simulink model "fft_test"  (R2019a)
settings: Solver=VariableStepDiscrete  StartTime=0.0  StopTime=50000  RelTol=1e-3
libraries: xbsIndex_r4 x4228, casper_library_misc x129, xps_library x1
(part 1 of 42)
settings Model: Creator=cicada  LastModifiedBy=kocz
settings SolverCC: ZeroCrossControl=EnableAll
settings DataIOCC: LimitDataPoints=on  SaveFormat=Array  SignalLoggingSaveFormat=ModelDataLogs  ReturnWorkspaceOutputs=off
settings OptimizationCC: DefaultParameterBehavior=Inlined  ExpressionDepthLimit=2147483647  LifeSpan=inf
settings DebuggingCC: WriteAfterWriteMsg=EnableAllAsError  SignalResolutionControl=TryResolveAllWithWarning  SolverPrmCheckMsg=warning  FcnCallInpInsideContextMsg=warning  StateNameClashWarn=warning  PregeneratedLibrarySubsystemCodeDiagnostic=none  StrictBusMsg=ErrorOnBusTreatedAsVector  SFUnexpectedBacktrackingDiag=warning  SFNoUnconditionalDefaultTransitionDiag=warning  SFExecutionAtInitializationDiag=none  ArithmeticOperatorsInVariantConditions=warning
settings HardwareCC: ProdBitPerPointer=32  ProdBitPerSizeT=32  ProdBitPerPtrDiffT=32  ProdLargestAtomicFloat=None  ProdIntDivRoundTo=Undefined  ProdEndianess=Unspecified  ProdWordSize=32  ProdHWDeviceType=32-bit Generic
settings ModelReferenceCC: PropagateSignalLabelsOutOfModel=off
settings SFSimCC: SimUseLocalCustomCode=off
settings RTWCC: RTWUseLocalCustomCode=off
settings CodeAppCC: StateflowObjectComments=on
settings GRTTargetCC: TargetLangStandard=C89/C90 (ANSI)  GeneratePreprocessorConditionals=Disable all  CombineOutputUpdateFcns=off  GRTInterface=on
settings ConfigComp: CovMetricSettings=dw  CovHtmlReporting=on  CovSaveCumulativeToWorkspaceVar=on  CovSaveSingleToWorkspaceVar=on  CovExternalEMLEnable=off

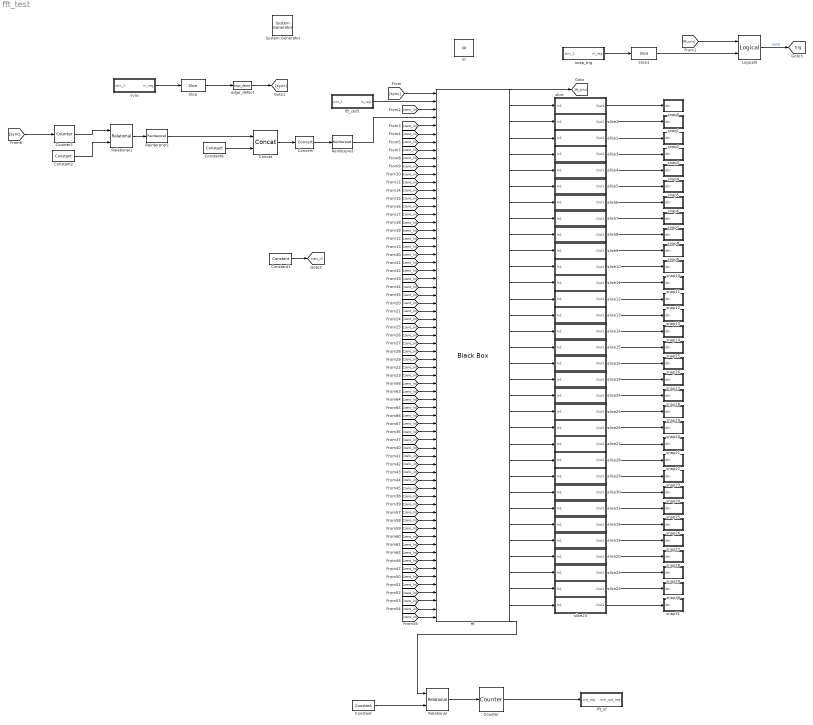
== system fft_test ==
  " System Generator" : xbsIndex_r4/ System Generator  Tag=genX  xilinxfamily=kintex7  part=xc7k325t  speed=-3  package=fbg676  synthesis_tool=Vivado  clock_wrapper=Clock Enables  directory=./netlist  proj_type=Vivado  Synth_file=Vivado Synthesis Defaults  Impl_file=Vivado Implementation Defaults  testbench=off  simulink_period=1  sysclk_period=10  dcm_input_clock_period=10  incr_netlist=off  trim_vbits=Everywhere in SubSystem  dbl_ovrd=According to Block Masks  core_generation=According to Block Masks  run_coregen=off  deprecated_control=off  eval_field=0  block_type=sysgen
  Concat : xbsIndex_r4/Concat  num_inputs=2  dbl_ovrd=off  block_type=concat
  Constant : xbsIndex_r4/Constant  const=0  gui_display_data_type=Fixed-point  arith_type=Unsigned  n_bits=16  bin_pt=0  preci_type=Single  exp_width=8  frac_width=24  explicit_period=on  period=1  equ=P=C  opselect=C  inp2=PCIN>>17  opr=+  inp1=P  carry=CIN  dbl_ovrd=off  block_type=constant
  Constant1 : xbsIndex_r4/Constant  const=0  gui_display_data_type=Fixed-point  arith_type=Signed (2's comp)  n_bits=18  bin_pt=17  preci_type=Single  exp_width=8  frac_width=24  explicit_period=on  period=1  equ=P=C  opselect=C  inp2=PCIN>>17  opr=+  inp1=P  carry=CIN  dbl_ovrd=off  block_type=constant
  Constant2 : xbsIndex_r4/Constant  const=1  gui_display_data_type=Fixed-point  arith_type=Unsigned  n_bits=32  bin_pt=0  preci_type=Single  exp_width=8  frac_width=24  explicit_period=on  period=1  equ=P=C  opselect=C  inp2=PCIN>>17  opr=+  inp1=P  carry=CIN  dbl_ovrd=off  block_type=constant
  Constant6 : xbsIndex_r4/Constant  const=0  gui_display_data_type=Fixed-point  arith_type=Unsigned  n_bits=4  bin_pt=0  preci_type=Single  exp_width=8  frac_width=24  explicit_period=on  period=1  equ=P=C  opselect=C  inp2=PCIN>>17  opr=+  inp1=P  carry=CIN  dbl_ovrd=off  block_type=constant
  Convert : xbsIndex_r4/Convert  gui_display_data_type=Fixed-point  arith_type=Unsigned  n_bits=18  bin_pt=0  float_type=Single  exp_bits=8  fraction_bits=24  quantization=Truncate  overflow=Wrap  en=off  latency=2  pipeline=off  dbl_ovrd=off  block_type=convert
  Counter : xbsIndex_r4/Counter  cnt_type=Free Running  cnt_to=Inf  operation=Up  start_count=0  cnt_by_val=1  arith_type=Unsigned  n_bits=16  bin_pt=0  load_pin=off  rst=off  en=on  explicit_period=on  period=1  use_behavioral_HDL=off  implementation=Fabric  dbl_ovrd=off  block_type=counter
  Counter1 : xbsIndex_r4/Counter  cnt_type=Free Running  cnt_to=Inf  operation=Up  start_count=0  cnt_by_val=1  arith_type=Unsigned  n_bits=12  bin_pt=0  load_pin=off  rst=on  en=off  explicit_period=on  period=1  use_behavioral_HDL=off  implementation=Fabric  dbl_ovrd=off  block_type=counter
  Logical5 : xbsIndex_r4/Logical  logical_function=AND  inputs=2  en=off  latency=1  precision=Full  arith_type=Unsigned  n_bits=16  bin_pt=0  align_bp=on  dbl_ovrd=off  block_type=logical
  Reinterpret : xbsIndex_r4/Reinterpret  force_arith_type=on  arith_type="Signed  (2's comp)"  force_bin_pt=on  bin_pt=17  block_type=reinterpret
  Reinterpret1 : xbsIndex_r4/Reinterpret  force_arith_type=on  arith_type=Unsigned  force_bin_pt=on  bin_pt=0  block_type=reinterpret
  Relational : xbsIndex_r4/Relational  mode=a>b  op_type=Bool  en=off  latency=1  dbl_ovrd=off  block_type=relational
  Relational1 : xbsIndex_r4/Relational  mode=a=b  op_type=Bool  en=off  latency=0  dbl_ovrd=off  block_type=relational
  Slice : xbsIndex_r4/Slice  nbits=1  boolean_output=on  mode=Lower Bit Location + Width  bit1=0  base1=MSB of Input  bit0=0  base0=LSB of Input  dbl_ovrd=off  block_type=slice
  Slice1 : xbsIndex_r4/Slice  nbits=1  boolean_output=on  mode=Lower Bit Location + Width  bit1=0  base1=MSB of Input  bit0=0  base0=LSB of Input  dbl_ovrd=off  block_type=slice
  edge_detect : casper_library_misc/edge_detect  edge=Rising  polarity=Active High  x_in=[0 0.08 0.08 0.16 0.16 0.24 0.24 0.32 0.32 0.4]  y_in="[-1 -1  1  1  1  1  1  1  1  1]"  x_out=[0.6 0.68 0.68 0.76 0.76 0.84 0.84 0.92 0.92 1]  y_out="[-1 -1  1  1 -1 -1 -1 -1 -1 -1]"
  fft : xbsIndex_r4/Black Box  init_code=fft_2019_rord_config  sim_method=ISE Simulator  verbose=off  block_type=blackbox2
  fft_of : Subsystem  Tag=xps:sw_reg  AncestorBlock=xps_library/Memory/software_register  mask(swreg){io_dir=To Processor, io_delay=0, init_val=0, sample_period=1, names=reg, bitwidths=16, bin_pts=0, arith_types=0, sim_port=on, show_format=on}
      mask prompts: io_dir "I/O direction"; io_delay "I/O delay"; init_val "Initial Value"; sample_period "Sample period"; names "Bitfield names [msb...lsb]"; bitwidths "Bitfield widths"; bin_pts "Bitfield binary pts"; arith_types "Bitfield types, ufix=0, fix=1, bool=2"; sim_port "Provide sim input/output?"; show_format "Print format string?"
      mask help: A 32-bit software-accessible register. Can be divided into bitfields of varying widths and types using the fields in the block mask.
      mask init:
      | swreg_init(gcb)
      settings: AttributesFormatString=1output:uf16.0 = 16 bits
      mask TypeOptions io_dir: To Processor | From Processor
      mask Callback io_dir:
      | mask_enables = get_param(gcb, 'MaskEnables');
      | mask_names = get_param(gcb, 'MaskNames');
      | if strcmp(get_param(gcb, 'io_dir'), 'To Processor'),
      |     mask_enables{ismember(mask_names, 'sample_period')} = 'off';
      | else
      |     mask_enables{ismember(mask_names, 'sample_period')} = 'on';
      | end
      | set_param(gcb, 'MaskEnables', mask_enables);
      mask DialogControl ParameterTabVar0 Prompt: Setup
  fft_shift : Subsystem  Tag=xps:sw_reg  AncestorBlock=xps_library/Memory/software_register  mask(swreg){io_dir=From Processor, io_delay=0, init_val=0, sample_period=1, names=reg, bitwidths=32, bin_pts=0, arith_types=0, sim_port=on, show_format=on}
      mask prompts: io_dir "I/O direction"; io_delay "I/O delay"; init_val "Initial Value"; sample_period "Sample period"; names "Bitfield names [msb...lsb]"; bitwidths "Bitfield widths"; bin_pts "Bitfield binary pts"; arith_types "Bitfield types, ufix=0, fix=1, bool=2"; sim_port "Provide sim input/output?"; show_format "Print format string?"
      mask help: A 32-bit software-accessible register. Can be divided into bitfields of varying widths and types using the fields in the block mask.
      mask init:
      | swreg_init(gcb)
      settings: AttributesFormatString=1input:uf32.0 = 32 bits
      mask TypeOptions io_dir: To Processor | From Processor
      mask Callback io_dir:
      | mask_enables = get_param(gcb, 'MaskEnables');
      | mask_names = get_param(gcb, 'MaskNames');
      | if strcmp(get_param(gcb, 'io_dir'), 'To Processor'),
      |     mask_enables{ismember(mask_names, 'sample_period')} = 'off';
      | else
      |     mask_enables{ismember(mask_names, 'sample_period')} = 'on';
      | end
      | set_param(gcb, 'MaskEnables', mask_enables);
      mask DialogControl ParameterTabVar0 Prompt: Setup
  ip : xps_library/Utilities/ip  Tag=xps:ip  lib_path=[fileparts(which(gcs)) '/fft_2019_default']  ip_name='fft_2019_default'
      settings: SourceProductName=CASPER XPS Blockset
  slice : Subsystem
  slice1 : Subsystem
  slice10 : Subsystem
  slice11 : Subsystem
  slice12 : Subsystem
  slice13 : Subsystem
  slice14 : Subsystem
  slice15 : Subsystem
  slice16 : Subsystem
  slice17 : Subsystem
  slice18 : Subsystem
  slice19 : Subsystem
  slice2 : Subsystem
  slice20 : Subsystem
  slice21 : Subsystem
  slice22 : Subsystem
  slice23 : Subsystem
  slice24 : Subsystem
  slice25 : Subsystem
  slice26 : Subsystem
  slice27 : Subsystem
  slice28 : Subsystem
  slice29 : Subsystem
  slice3 : Subsystem
  slice30 : Subsystem
  slice31 : Subsystem
  slice4 : Subsystem
  slice5 : Subsystem
  slice6 : Subsystem
  slice7 : Subsystem
  slice8 : Subsystem
  slice9 : Subsystem
  snap0 : Subsystem
  snap1 : Subsystem
  snap10 : Subsystem
  snap11 : Subsystem
  snap12 : Subsystem
  snap13 : Subsystem
  snap14 : Subsystem
  snap15 : Subsystem
  snap16 : Subsystem
  snap17 : Subsystem
  snap18 : Subsystem
  snap19 : Subsystem
  snap2 : Subsystem
  snap20 : Subsystem
  snap21 : Subsystem
  snap22 : Subsystem
  snap23 : Subsystem
  snap24 : Subsystem
  snap25 : Subsystem
  snap26 : Subsystem
  snap27 : Subsystem
  snap28 : Subsystem
  snap29 : Subsystem
  snap3 : Subsystem
  snap30 : Subsystem
  snap31 : Subsystem
  snap4 : Subsystem
  snap5 : Subsystem
  snap6 : Subsystem
  snap7 : Subsystem
  snap8 : Subsystem
  snap9 : Subsystem
  snap_trig : Subsystem  Tag=xps:sw_reg  AncestorBlock=xps_library/Memory/software_register  mask(swreg){io_dir=From Processor, io_delay=0, init_val=0, sample_period=1, names=reg, bitwidths=32, bin_pts=0, arith_types=0, sim_port=on, show_format=on}
      mask prompts: io_dir "I/O direction"; io_delay "I/O delay"; init_val "Initial Value"; sample_period "Sample period"; names "Bitfield names [msb...lsb]"; bitwidths "Bitfield widths"; bin_pts "Bitfield binary pts"; arith_types "Bitfield types, ufix=0, fix=1, bool=2"; sim_port "Provide sim input/output?"; show_format "Print format string?"
      mask help: A 32-bit software-accessible register. Can be divided into bitfields of varying widths and types using the fields in the block mask.
      mask init:
      | swreg_init(gcb)
      settings: AttributesFormatString=1input:uf32.0 = 32 bits
      mask TypeOptions io_dir: To Processor | From Processor
      mask Callback io_dir:
      | mask_enables = get_param(gcb, 'MaskEnables');
      | mask_names = get_param(gcb, 'MaskNames');
      | if strcmp(get_param(gcb, 'io_dir'), 'To Processor'),
      |     mask_enables{ismember(mask_names, 'sample_period')} = 'off';
      | else
      |     mask_enables{ismember(mask_names, 'sample_period')} = 'on';
      | end
      | set_param(gcb, 'MaskEnables', mask_enables);
      mask DialogControl ParameterTabVar0 Prompt: Setup
  sync : Subsystem  Tag=xps:sw_reg  AncestorBlock=xps_library/Memory/software_register  mask(swreg){io_dir=From Processor, io_delay=0, init_val=0, sample_period=1, names=reg, bitwidths=32, bin_pts=0, arith_types=0, sim_port=on, show_format=on}
      mask prompts: io_dir "I/O direction"; io_delay "I/O delay"; init_val "Initial Value"; sample_period "Sample period"; names "Bitfield names [msb...lsb]"; bitwidths "Bitfield widths"; bin_pts "Bitfield binary pts"; arith_types "Bitfield types, ufix=0, fix=1, bool=2"; sim_port "Provide sim input/output?"; show_format "Print format string?"
      mask help: A 32-bit software-accessible register. Can be divided into bitfields of varying widths and types using the fields in the block mask.
      mask init:
      | swreg_init(gcb)
      settings: AttributesFormatString=1input:uf32.0 = 32 bits
      mask TypeOptions io_dir: To Processor | From Processor
      mask Callback io_dir:
      | mask_enables = get_param(gcb, 'MaskEnables');
      | mask_names = get_param(gcb, 'MaskNames');
      | if strcmp(get_param(gcb, 'io_dir'), 'To Processor'),
      |     mask_enables{ismember(mask_names, 'sample_period')} = 'off';
      | else
      |     mask_enables{ismember(mask_names, 'sample_period')} = 'on';
      | end
      | set_param(gcb, 'MaskEnables', mask_enables);
      mask DialogControl ParameterTabVar0 Prompt: Setup
  tag scope: trig=global
  wires:
  fft_shift/1(in_reg) -> fft/2
  fft/1 -> [fft_sync]
  Relational/1 -> Counter/1
  Constant/1 -> Relational/2
  fft/34 -> Relational/1
  Counter/1 -> fft_of/1(out_reg)
  Slice/1 -> edge_detect/1
  sync/1(in_reg) -> Slice/1
  Constant6/1 -> Concat/2
  Reinterpret1/1 -> Concat/1
  Relational1/1 -> Reinterpret1/1
  Concat/1 -> Convert/1
  Convert/1 -> Reinterpret/1
  Constant2/1 -> Relational1/2
  Counter1/1 -> Relational1/1
  Reinterpret/1 -> fft/4
  edge_detect/1 -> [sync]
  Constant1/1 -> [zero_in]
  [zero_in] -> fft/3
  [zero_in] -> fft/5
  [zero_in] -> fft/6
  [zero_in] -> fft/7
  [sync] -> fft/1
  [sync] -> Counter1/1
  [zero_in] -> fft/8
  [zero_in] -> fft/12
  [zero_in] -> fft/11
  [zero_in] -> fft/10
  [zero_in] -> fft/9
  [zero_in] -> fft/17
  [zero_in] -> fft/18
  [zero_in] -> fft/19
  [zero_in] -> fft/20
  [zero_in] -> fft/16
  [zero_in] -> fft/15
  [zero_in] -> fft/14
  [zero_in] -> fft/13
  [zero_in] -> fft/29
  [zero_in] -> fft/30
  [zero_in] -> fft/31
  [zero_in] -> fft/32
  [zero_in] -> fft/36
  [zero_in] -> fft/35
  [zero_in] -> fft/34
  [zero_in] -> fft/33
  [zero_in] -> fft/25
  [zero_in] -> fft/26
  [zero_in] -> fft/27
  [zero_in] -> fft/28
  [zero_in] -> fft/24
  [zero_in] -> fft/23
  [zero_in] -> fft/22
  [zero_in] -> fft/21
  [zero_in] -> fft/53
  [zero_in] -> fft/54
  [zero_in] -> fft/55
  [zero_in] -> fft/56
  [zero_in] -> fft/60
  [zero_in] -> fft/59
  [zero_in] -> fft/58
  [zero_in] -> fft/57
  [zero_in] -> fft/65
  [zero_in] -> fft/66
  [zero_in] -> fft/64
  [zero_in] -> fft/63
  [zero_in] -> fft/62
  [zero_in] -> fft/61
  [zero_in] -> fft/45
  [zero_in] -> fft/46
  [zero_in] -> fft/47
  [zero_in] -> fft/48
  [zero_in] -> fft/52
  [zero_in] -> fft/51
  [zero_in] -> fft/50
  [zero_in] -> fft/49
  [zero_in] -> fft/41
  [zero_in] -> fft/42
  [zero_in] -> fft/43
  [zero_in] -> fft/44
  [zero_in] -> fft/40
  [zero_in] -> fft/39
  [zero_in] -> fft/38
  [zero_in] -> fft/37
  fft/2 -> slice/1(In1)
  fft/3 -> slice1/1(In1)
  fft/4 -> slice2/1(In1)
  fft/5 -> slice3/1(In1)
  fft/6 -> slice4/1(In1)
  fft/7 -> slice5/1(In1)
  fft/8 -> slice6/1(In1)
  fft/9 -> slice7/1(In1)
  fft/10 -> slice8/1(In1)
  fft/11 -> slice9/1(In1)
  fft/12 -> slice10/1(In1)
  fft/13 -> slice11/1(In1)
  fft/14 -> slice12/1(In1)
  fft/15 -> slice13/1(In1)
  fft/16 -> slice14/1(In1)
  fft/17 -> slice15/1(In1)
  fft/18 -> slice16/1(In1)
  fft/19 -> slice17/1(In1)
  fft/20 -> slice24/1(In1)
  fft/21 -> slice25/1(In1)
  fft/22 -> slice26/1(In1)
  fft/23 -> slice27/1(In1)
  fft/24 -> slice28/1(In1)
  fft/25 -> slice29/1(In1)
  fft/26 -> slice30/1(In1)
  fft/27 -> slice31/1(In1)
  fft/28 -> slice18/1(In1)
  fft/29 -> slice19/1(In1)
  fft/30 -> slice20/1(In1)
  fft/31 -> slice21/1(In1)
  fft/32 -> slice22/1(In1)
  fft/33 -> slice23/1(In1)
  slice/1(Out1) -> snap0/1(din)
  slice1/1(Out1) -> snap1/1(din)
  slice3/1(Out1) -> snap3/1(din)
  slice2/1(Out1) -> snap2/1(din)
  slice5/1(Out1) -> snap5/1(din)
  slice7/1(Out1) -> snap7/1(din)
  slice6/1(Out1) -> snap6/1(din)
  slice4/1(Out1) -> snap4/1(din)
  slice12/1(Out1) -> snap12/1(din)
  slice11/1(Out1) -> snap11/1(din)
  slice15/1(Out1) -> snap15/1(din)
  slice8/1(Out1) -> snap8/1(din)
  slice9/1(Out1) -> snap9/1(din)
  slice13/1(Out1) -> snap13/1(din)
  slice10/1(Out1) -> snap10/1(din)
  slice14/1(Out1) -> snap14/1(din)
  slice18/1(Out1) -> snap26/1(din)
  slice16/1(Out1) -> snap16/1(din)
  slice27/1(Out1) -> snap21/1(din)
  slice21/1(Out1) -> snap29/1(din)
  slice28/1(Out1) -> snap22/1(din)
  slice29/1(Out1) -> snap23/1(din)
  slice26/1(Out1) -> snap20/1(din)
  slice22/1(Out1) -> snap30/1(din)
  slice23/1(Out1) -> snap31/1(din)
  slice31/1(Out1) -> snap25/1(din)
  slice25/1(Out1) -> snap19/1(din)
  slice30/1(Out1) -> snap24/1(din)
  slice17/1(Out1) -> snap17/1(din)
  slice20/1(Out1) -> snap28/1(din)
  slice19/1(Out1) -> snap27/1(din)
  slice24/1(Out1) -> snap18/1(din)
  [fft_sync] -> Logical5/1
  snap_trig/1(in_reg) -> Slice1/1
  Slice1/1 -> Logical5/2
  Logical5/1 -> [trig]  "valid"

== system fft_test/fft_of ==
  out_reg : Inport
  assert_reg : xbsIndex_r4/Assert  assert_type=on  type_source=Explicitly  gui_display_data_type=Fixed-point  arith_type=Unsigned  n_bits=16  bin_pt=0  preci_type=Single  exp_width=8  frac_width=24  assert_rate=off  rate_source=Explicitly  period=1  output_port=on  block_type=assert
  cast_gw : xbsIndex_r4/Convert  gui_display_data_type=Fixed-point  arith_type=Unsigned  n_bits=32  bin_pt=0  float_type=Single  exp_bits=8  fraction_bits=24  quantization=Truncate  overflow=Wrap  en=off  latency=1  pipeline=off  dbl_ovrd=off  block_type=convert
  fft_test_fft_of_user_data_in : xbsIndex_r4/Gateway Out  inherit_from_input=off  hdl_port=on  rows=1  columns=1  UseAsDAC=off  DACChannel='1'  interface=None  automatic_assignment=on  address_offset=hex2dec('00')  intf_name=''  intf_description=''  timing_constraint=None  locs_specified=off  LOCs={}  io_standard={}  block_type=gatewayout
  io_delay : xbsIndex_r4/Delay  rst=off  infoeditControl=Selection of Reset will increase slice count due to use of real FFs and instead of SRLs  en=off  latency=0  reg_retiming=on  dbl_ovrd=off  block_type=delay
  reint1 : xbsIndex_r4/Reinterpret  force_arith_type=on  arith_type=Unsigned  force_bin_pt=on  bin_pt=0  block_type=reinterpret
  sim_out : Terminator
  sim_out_reg_gw : xbsIndex_r4/Gateway Out  inherit_from_input=off  hdl_port=off  rows=1  columns=1  UseAsDAC=off  DACChannel='1'  interface=None  automatic_assignment=on  address_offset=hex2dec('00')  intf_name=''  intf_description=''  timing_constraint=None  locs_specified=off  LOCs={}  io_standard={}  block_type=gatewayout
  sim_out_reg_sim_delay : xbsIndex_r4/Delay  rst=off  infoeditControl=Selection of Reset will increase slice count due to use of real FFs and instead of SRLs  en=off  latency=1  reg_retiming=on  dbl_ovrd=off  block_type=delay
  sim_out_reg : Outport
  wires:
  sim_out_reg_sim_delay/1 -> sim_out_reg_gw/1
  sim_out_reg_gw/1 -> sim_out_reg/1
  io_delay/1 -> cast_gw/1
  cast_gw/1 -> fft_test_fft_of_user_data_in/1
  fft_test_fft_of_user_data_in/1 -> sim_out/1
  out_reg/1 -> sim_out_reg_sim_delay/1, assert_reg/1
  assert_reg/1 -> reint1/1
  reint1/1 -> io_delay/1

== system fft_test/fft_shift ==
  sim_1 : Inport
  convert1_1 : DataTypeConversion  OutDataTypeStr=fixdt('ufix32_En0')  LockScale=on
  convert2_1 : DataTypeConversion  OutDataTypeStr=fixdt('ufix32_En0')  ConvertRealWorld=Stored Integer (SI)  LockScale=on
  fft_test_fft_shift_user_data_out : xbsIndex_r4/Gateway In  gui_display_data_type=Fixed-point  arith_type=Unsigned  n_bits=32  bin_pt=0  preci_type=Single  exp_width=8  frac_width=24  rows=1  columns=1  quantization="Round  (unbiased: +/- Inf)"  overflow=Saturate  period=1  UseAsADC=off  ADCChannel='1'  interface=None  automatic_assignment=on  address_offset=hex2dec('00')  intf_name=''  intf_description=''  default_value=0  timing_constraint=None  locs_specified=off  LOCs={}  io_standard={}  inherit_from_input=off  hdl_port=on  dbl_ovrd=off  block_type=gatewayin
  gain_1 : Gain
  io_delay : xbsIndex_r4/Delay  rst=off  infoeditControl=Selection of Reset will increase slice count due to use of real FFs and instead of SRLs  en=off  latency=0  reg_retiming=on  dbl_ovrd=off  block_type=delay
  reint1 : xbsIndex_r4/Reinterpret  force_arith_type=on  arith_type=Unsigned  force_bin_pt=on  bin_pt=0  block_type=reinterpret
  slice_reg : xbsIndex_r4/Slice  nbits=32  boolean_output=off  mode=Lower Bit Location + Width  bit1=0  base1=MSB of Input  bit0=0  base0=LSB of Input  dbl_ovrd=off  block_type=slice
  in_reg : Outport
  wires:
  fft_test_fft_shift_user_data_out/1 -> io_delay/1
  sim_1/1 -> convert1_1/1
  convert1_1/1 -> convert2_1/1
  convert2_1/1 -> gain_1/1
  gain_1/1 -> fft_test_fft_shift_user_data_out/1
  io_delay/1 -> slice_reg/1
  slice_reg/1 -> reint1/1
  reint1/1 -> in_reg/1

== system fft_test/slice ==
  In1 : Inport
  Slice1 : xbsIndex_r4/Slice  nbits=16  boolean_output=off  mode=Upper Bit Location + Width  bit1=0  base1=MSB of Input  bit0=0  base0=LSB of Input  dbl_ovrd=off  block_type=slice
  Slice2 : xbsIndex_r4/Slice  nbits=16  boolean_output=off  mode=Upper Bit Location + Width  bit1=0  base1=MSB of Input  bit0=0  base0=LSB of Input  dbl_ovrd=off  block_type=slice
  c_to_ri : casper_library_misc/c_to_ri  n_bits=8  bin_pt=7
      settings: AttributesFormatString=8_7 r/i  SourceProductName=CASPER DSP Blockset
  ri_to_c : casper_library_misc/ri_to_c
      settings: SourceProductName=CASPER DSP Blockset
  Out1 : Outport
  wires:
  Slice1/1 -> ri_to_c/1
  In1/1 -> c_to_ri/1
  Slice2/1 -> ri_to_c/2
  c_to_ri/1 -> Slice1/1
  ri_to_c/1 -> Out1/1
  c_to_ri/2 -> Slice2/1

== system fft_test/slice1 ==
  In1 : Inport
  Slice1 : xbsIndex_r4/Slice  nbits=16  boolean_output=off  mode=Upper Bit Location + Width  bit1=0  base1=MSB of Input  bit0=0  base0=LSB of Input  dbl_ovrd=off  block_type=slice
  Slice2 : xbsIndex_r4/Slice  nbits=16  boolean_output=off  mode=Upper Bit Location + Width  bit1=0  base1=MSB of Input  bit0=0  base0=LSB of Input  dbl_ovrd=off  block_type=slice
  c_to_ri : casper_library_misc/c_to_ri  n_bits=8  bin_pt=7
      settings: AttributesFormatString=8_7 r/i  SourceProductName=CASPER DSP Blockset
  ri_to_c : casper_library_misc/ri_to_c
      settings: SourceProductName=CASPER DSP Blockset
  Out1 : Outport
  wires:
  c_to_ri/2 -> Slice2/1
  ri_to_c/1 -> Out1/1
  c_to_ri/1 -> Slice1/1
  Slice2/1 -> ri_to_c/2
  In1/1 -> c_to_ri/1
  Slice1/1 -> ri_to_c/1

== system fft_test/slice10 ==
  In1 : Inport
  Slice1 : xbsIndex_r4/Slice  nbits=16  boolean_output=off  mode=Upper Bit Location + Width  bit1=0  base1=MSB of Input  bit0=0  base0=LSB of Input  dbl_ovrd=off  block_type=slice
  Slice2 : xbsIndex_r4/Slice  nbits=16  boolean_output=off  mode=Upper Bit Location + Width  bit1=0  base1=MSB of Input  bit0=0  base0=LSB of Input  dbl_ovrd=off  block_type=slice
  c_to_ri : casper_library_misc/c_to_ri  n_bits=8  bin_pt=7
      settings: AttributesFormatString=8_7 r/i  SourceProductName=CASPER DSP Blockset
  ri_to_c : casper_library_misc/ri_to_c
      settings: SourceProductName=CASPER DSP Blockset
  Out1 : Outport
  wires:
  Slice1/1 -> ri_to_c/1
  In1/1 -> c_to_ri/1
  Slice2/1 -> ri_to_c/2
  c_to_ri/1 -> Slice1/1
  ri_to_c/1 -> Out1/1
  c_to_ri/2 -> Slice2/1

== system fft_test/slice11 ==
  In1 : Inport
  Slice1 : xbsIndex_r4/Slice  nbits=16  boolean_output=off  mode=Upper Bit Location + Width  bit1=0  base1=MSB of Input  bit0=0  base0=LSB of Input  dbl_ovrd=off  block_type=slice
  Slice2 : xbsIndex_r4/Slice  nbits=16  boolean_output=off  mode=Upper Bit Location + Width  bit1=0  base1=MSB of Input  bit0=0  base0=LSB of Input  dbl_ovrd=off  block_type=slice
  c_to_ri : casper_library_misc/c_to_ri  n_bits=8  bin_pt=7
      settings: AttributesFormatString=8_7 r/i  SourceProductName=CASPER DSP Blockset
  ri_to_c : casper_library_misc/ri_to_c
      settings: SourceProductName=CASPER DSP Blockset
  Out1 : Outport
  wires:
  c_to_ri/2 -> Slice2/1
  ri_to_c/1 -> Out1/1
  c_to_ri/1 -> Slice1/1
  Slice2/1 -> ri_to_c/2
  In1/1 -> c_to_ri/1
  Slice1/1 -> ri_to_c/1

== system fft_test/slice12 ==
  In1 : Inport
  Slice1 : xbsIndex_r4/Slice  nbits=16  boolean_output=off  mode=Upper Bit Location + Width  bit1=0  base1=MSB of Input  bit0=0  base0=LSB of Input  dbl_ovrd=off  block_type=slice
  Slice2 : xbsIndex_r4/Slice  nbits=16  boolean_output=off  mode=Upper Bit Location + Width  bit1=0  base1=MSB of Input  bit0=0  base0=LSB of Input  dbl_ovrd=off  block_type=slice
  c_to_ri : casper_library_misc/c_to_ri  n_bits=8  bin_pt=7
      settings: AttributesFormatString=8_7 r/i  SourceProductName=CASPER DSP Blockset
  ri_to_c : casper_library_misc/ri_to_c
      settings: SourceProductName=CASPER DSP Blockset
  Out1 : Outport
  wires:
  Slice1/1 -> ri_to_c/1
  In1/1 -> c_to_ri/1
  Slice2/1 -> ri_to_c/2
  c_to_ri/1 -> Slice1/1
  ri_to_c/1 -> Out1/1
  c_to_ri/2 -> Slice2/1

== system fft_test/slice13 ==
  In1 : Inport
  Slice1 : xbsIndex_r4/Slice  nbits=16  boolean_output=off  mode=Upper Bit Location + Width  bit1=0  base1=MSB of Input  bit0=0  base0=LSB of Input  dbl_ovrd=off  block_type=slice
  Slice2 : xbsIndex_r4/Slice  nbits=16  boolean_output=off  mode=Upper Bit Location + Width  bit1=0  base1=MSB of Input  bit0=0  base0=LSB of Input  dbl_ovrd=off  block_type=slice
  c_to_ri : casper_library_misc/c_to_ri  n_bits=8  bin_pt=7
      settings: AttributesFormatString=8_7 r/i  SourceProductName=CASPER DSP Blockset
  ri_to_c : casper_library_misc/ri_to_c
      settings: SourceProductName=CASPER DSP Blockset
  Out1 : Outport
  wires:
  c_to_ri/2 -> Slice2/1
  ri_to_c/1 -> Out1/1
  c_to_ri/1 -> Slice1/1
  Slice2/1 -> ri_to_c/2
  In1/1 -> c_to_ri/1
  Slice1/1 -> ri_to_c/1

== system fft_test/slice14 ==
  In1 : Inport
  Slice1 : xbsIndex_r4/Slice  nbits=16  boolean_output=off  mode=Upper Bit Location + Width  bit1=0  base1=MSB of Input  bit0=0  base0=LSB of Input  dbl_ovrd=off  block_type=slice
  Slice2 : xbsIndex_r4/Slice  nbits=16  boolean_output=off  mode=Upper Bit Location + Width  bit1=0  base1=MSB of Input  bit0=0  base0=LSB of Input  dbl_ovrd=off  block_type=slice
  c_to_ri : casper_library_misc/c_to_ri  n_bits=8  bin_pt=7
      settings: AttributesFormatString=8_7 r/i  SourceProductName=CASPER DSP Blockset
  ri_to_c : casper_library_misc/ri_to_c
      settings: SourceProductName=CASPER DSP Blockset
  Out1 : Outport
  wires:
  c_to_ri/2 -> Slice2/1
  ri_to_c/1 -> Out1/1
  c_to_ri/1 -> Slice1/1
  Slice2/1 -> ri_to_c/2
  In1/1 -> c_to_ri/1
  Slice1/1 -> ri_to_c/1

== system fft_test/slice15 ==
  In1 : Inport
  Slice1 : xbsIndex_r4/Slice  nbits=16  boolean_output=off  mode=Upper Bit Location + Width  bit1=0  base1=MSB of Input  bit0=0  base0=LSB of Input  dbl_ovrd=off  block_type=slice
  Slice2 : xbsIndex_r4/Slice  nbits=16  boolean_output=off  mode=Upper Bit Location + Width  bit1=0  base1=MSB of Input  bit0=0  base0=LSB of Input  dbl_ovrd=off  block_type=slice
  c_to_ri : casper_library_misc/c_to_ri  n_bits=8  bin_pt=7
      settings: AttributesFormatString=8_7 r/i  SourceProductName=CASPER DSP Blockset
  ri_to_c : casper_library_misc/ri_to_c
      settings: SourceProductName=CASPER DSP Blockset
  Out1 : Outport
  wires:
  Slice1/1 -> ri_to_c/1
  In1/1 -> c_to_ri/1
  Slice2/1 -> ri_to_c/2
  c_to_ri/1 -> Slice1/1
  ri_to_c/1 -> Out1/1
  c_to_ri/2 -> Slice2/1

== system fft_test/slice16 ==
  In1 : Inport
  Slice1 : xbsIndex_r4/Slice  nbits=16  boolean_output=off  mode=Upper Bit Location + Width  bit1=0  base1=MSB of Input  bit0=0  base0=LSB of Input  dbl_ovrd=off  block_type=slice
  Slice2 : xbsIndex_r4/Slice  nbits=16  boolean_output=off  mode=Upper Bit Location + Width  bit1=0  base1=MSB of Input  bit0=0  base0=LSB of Input  dbl_ovrd=off  block_type=slice
  c_to_ri : casper_library_misc/c_to_ri  n_bits=8  bin_pt=7
      settings: AttributesFormatString=8_7 r/i  SourceProductName=CASPER DSP Blockset
  ri_to_c : casper_library_misc/ri_to_c
      settings: SourceProductName=CASPER DSP Blockset
  Out1 : Outport
  wires:
  c_to_ri/2 -> Slice2/1
  ri_to_c/1 -> Out1/1
  c_to_ri/1 -> Slice1/1
  Slice2/1 -> ri_to_c/2
  In1/1 -> c_to_ri/1
  Slice1/1 -> ri_to_c/1

== system fft_test/slice17 ==
  In1 : Inport
  Slice1 : xbsIndex_r4/Slice  nbits=16  boolean_output=off  mode=Upper Bit Location + Width  bit1=0  base1=MSB of Input  bit0=0  base0=LSB of Input  dbl_ovrd=off  block_type=slice
  Slice2 : xbsIndex_r4/Slice  nbits=16  boolean_output=off  mode=Upper Bit Location + Width  bit1=0  base1=MSB of Input  bit0=0  base0=LSB of Input  dbl_ovrd=off  block_type=slice
  c_to_ri : casper_library_misc/c_to_ri  n_bits=8  bin_pt=7
      settings: AttributesFormatString=8_7 r/i  SourceProductName=CASPER DSP Blockset
  ri_to_c : casper_library_misc/ri_to_c
      settings: SourceProductName=CASPER DSP Blockset
  Out1 : Outport
  wires:
  Slice1/1 -> ri_to_c/1
  In1/1 -> c_to_ri/1
  Slice2/1 -> ri_to_c/2
  c_to_ri/1 -> Slice1/1
  ri_to_c/1 -> Out1/1
  c_to_ri/2 -> Slice2/1

== system fft_test/slice18 ==
  In1 : Inport
  Slice1 : xbsIndex_r4/Slice  nbits=16  boolean_output=off  mode=Upper Bit Location + Width  bit1=0  base1=MSB of Input  bit0=0  base0=LSB of Input  dbl_ovrd=off  block_type=slice
  Slice2 : xbsIndex_r4/Slice  nbits=16  boolean_output=off  mode=Upper Bit Location + Width  bit1=0  base1=MSB of Input  bit0=0  base0=LSB of Input  dbl_ovrd=off  block_type=slice
  c_to_ri : casper_library_misc/c_to_ri  n_bits=8  bin_pt=7
      settings: AttributesFormatString=8_7 r/i  SourceProductName=CASPER DSP Blockset
  ri_to_c : casper_library_misc/ri_to_c
      settings: SourceProductName=CASPER DSP Blockset
  Out1 : Outport
  wires:
  c_to_ri/2 -> Slice2/1
  ri_to_c/1 -> Out1/1
  c_to_ri/1 -> Slice1/1
  Slice2/1 -> ri_to_c/2
  In1/1 -> c_to_ri/1
  Slice1/1 -> ri_to_c/1

== system fft_test/slice19 ==
  In1 : Inport
  Slice1 : xbsIndex_r4/Slice  nbits=16  boolean_output=off  mode=Upper Bit Location + Width  bit1=0  base1=MSB of Input  bit0=0  base0=LSB of Input  dbl_ovrd=off  block_type=slice
  Slice2 : xbsIndex_r4/Slice  nbits=16  boolean_output=off  mode=Upper Bit Location + Width  bit1=0  base1=MSB of Input  bit0=0  base0=LSB of Input  dbl_ovrd=off  block_type=slice
  c_to_ri : casper_library_misc/c_to_ri  n_bits=8  bin_pt=7
      settings: AttributesFormatString=8_7 r/i  SourceProductName=CASPER DSP Blockset
  ri_to_c : casper_library_misc/ri_to_c
      settings: SourceProductName=CASPER DSP Blockset
  Out1 : Outport
  wires:
  Slice1/1 -> ri_to_c/1
  In1/1 -> c_to_ri/1
  Slice2/1 -> ri_to_c/2
  c_to_ri/1 -> Slice1/1
  ri_to_c/1 -> Out1/1
  c_to_ri/2 -> Slice2/1

== system fft_test/slice2 ==
  In1 : Inport
  Slice1 : xbsIndex_r4/Slice  nbits=16  boolean_output=off  mode=Upper Bit Location + Width  bit1=0  base1=MSB of Input  bit0=0  base0=LSB of Input  dbl_ovrd=off  block_type=slice
  Slice2 : xbsIndex_r4/Slice  nbits=16  boolean_output=off  mode=Upper Bit Location + Width  bit1=0  base1=MSB of Input  bit0=0  base0=LSB of Input  dbl_ovrd=off  block_type=slice
  c_to_ri : casper_library_misc/c_to_ri  n_bits=8  bin_pt=7
      settings: AttributesFormatString=8_7 r/i  SourceProductName=CASPER DSP Blockset
  ri_to_c : casper_library_misc/ri_to_c
      settings: SourceProductName=CASPER DSP Blockset
  Out1 : Outport
  wires:
  c_to_ri/2 -> Slice2/1
  ri_to_c/1 -> Out1/1
  c_to_ri/1 -> Slice1/1
  Slice2/1 -> ri_to_c/2
  In1/1 -> c_to_ri/1
  Slice1/1 -> ri_to_c/1

== system fft_test/slice20 ==
  In1 : Inport
  Slice1 : xbsIndex_r4/Slice  nbits=16  boolean_output=off  mode=Upper Bit Location + Width  bit1=0  base1=MSB of Input  bit0=0  base0=LSB of Input  dbl_ovrd=off  block_type=slice
  Slice2 : xbsIndex_r4/Slice  nbits=16  boolean_output=off  mode=Upper Bit Location + Width  bit1=0  base1=MSB of Input  bit0=0  base0=LSB of Input  dbl_ovrd=off  block_type=slice
  c_to_ri : casper_library_misc/c_to_ri  n_bits=8  bin_pt=7
      settings: AttributesFormatString=8_7 r/i  SourceProductName=CASPER DSP Blockset
  ri_to_c : casper_library_misc/ri_to_c
      settings: SourceProductName=CASPER DSP Blockset
  Out1 : Outport
  wires:
  c_to_ri/2 -> Slice2/1
  ri_to_c/1 -> Out1/1
  c_to_ri/1 -> Slice1/1
  Slice2/1 -> ri_to_c/2
  In1/1 -> c_to_ri/1
  Slice1/1 -> ri_to_c/1

== system fft_test/slice21 ==
  In1 : Inport
  Slice1 : xbsIndex_r4/Slice  nbits=16  boolean_output=off  mode=Upper Bit Location + Width  bit1=0  base1=MSB of Input  bit0=0  base0=LSB of Input  dbl_ovrd=off  block_type=slice
  Slice2 : xbsIndex_r4/Slice  nbits=16  boolean_output=off  mode=Upper Bit Location + Width  bit1=0  base1=MSB of Input  bit0=0  base0=LSB of Input  dbl_ovrd=off  block_type=slice
  c_to_ri : casper_library_misc/c_to_ri  n_bits=8  bin_pt=7
      settings: AttributesFormatString=8_7 r/i  SourceProductName=CASPER DSP Blockset
  ri_to_c : casper_library_misc/ri_to_c
      settings: SourceProductName=CASPER DSP Blockset
  Out1 : Outport
  wires:
  Slice1/1 -> ri_to_c/1
  In1/1 -> c_to_ri/1
  Slice2/1 -> ri_to_c/2
  c_to_ri/1 -> Slice1/1
  ri_to_c/1 -> Out1/1
  c_to_ri/2 -> Slice2/1

== system fft_test/slice22 ==
  In1 : Inport
  Slice1 : xbsIndex_r4/Slice  nbits=16  boolean_output=off  mode=Upper Bit Location + Width  bit1=0  base1=MSB of Input  bit0=0  base0=LSB of Input  dbl_ovrd=off  block_type=slice
  Slice2 : xbsIndex_r4/Slice  nbits=16  boolean_output=off  mode=Upper Bit Location + Width  bit1=0  base1=MSB of Input  bit0=0  base0=LSB of Input  dbl_ovrd=off  block_type=slice
  c_to_ri : casper_library_misc/c_to_ri  n_bits=8  bin_pt=7
      settings: AttributesFormatString=8_7 r/i  SourceProductName=CASPER DSP Blockset
  ri_to_c : casper_library_misc/ri_to_c
      settings: SourceProductName=CASPER DSP Blockset
  Out1 : Outport
  wires:
  Slice1/1 -> ri_to_c/1
  In1/1 -> c_to_ri/1
  Slice2/1 -> ri_to_c/2
  c_to_ri/1 -> Slice1/1
  ri_to_c/1 -> Out1/1
  c_to_ri/2 -> Slice2/1

== system fft_test/slice23 ==
  In1 : Inport
  Slice1 : xbsIndex_r4/Slice  nbits=16  boolean_output=off  mode=Upper Bit Location + Width  bit1=0  base1=MSB of Input  bit0=0  base0=LSB of Input  dbl_ovrd=off  block_type=slice
  Slice2 : xbsIndex_r4/Slice  nbits=16  boolean_output=off  mode=Upper Bit Location + Width  bit1=0  base1=MSB of Input  bit0=0  base0=LSB of Input  dbl_ovrd=off  block_type=slice
  c_to_ri : casper_library_misc/c_to_ri  n_bits=8  bin_pt=7
      settings: AttributesFormatString=8_7 r/i  SourceProductName=CASPER DSP Blockset
  ri_to_c : casper_library_misc/ri_to_c
      settings: SourceProductName=CASPER DSP Blockset
  Out1 : Outport
  wires:
  c_to_ri/2 -> Slice2/1
  ri_to_c/1 -> Out1/1
  c_to_ri/1 -> Slice1/1
  Slice2/1 -> ri_to_c/2
  In1/1 -> c_to_ri/1
  Slice1/1 -> ri_to_c/1

== system fft_test/slice24 ==
  In1 : Inport
  Slice1 : xbsIndex_r4/Slice  nbits=16  boolean_output=off  mode=Upper Bit Location + Width  bit1=0  base1=MSB of Input  bit0=0  base0=LSB of Input  dbl_ovrd=off  block_type=slice
  Slice2 : xbsIndex_r4/Slice  nbits=16  boolean_output=off  mode=Upper Bit Location + Width  bit1=0  base1=MSB of Input  bit0=0  base0=LSB of Input  dbl_ovrd=off  block_type=slice
  c_to_ri : casper_library_misc/c_to_ri  n_bits=8  bin_pt=7
      settings: AttributesFormatString=8_7 r/i  SourceProductName=CASPER DSP Blockset
  ri_to_c : casper_library_misc/ri_to_c
      settings: SourceProductName=CASPER DSP Blockset
  Out1 : Outport
  wires:
  Slice1/1 -> ri_to_c/1
  In1/1 -> c_to_ri/1
  Slice2/1 -> ri_to_c/2
  c_to_ri/1 -> Slice1/1
  ri_to_c/1 -> Out1/1
  c_to_ri/2 -> Slice2/1

== system fft_test/slice25 ==
  In1 : Inport
  Slice1 : xbsIndex_r4/Slice  nbits=16  boolean_output=off  mode=Upper Bit Location + Width  bit1=0  base1=MSB of Input  bit0=0  base0=LSB of Input  dbl_ovrd=off  block_type=slice
  Slice2 : xbsIndex_r4/Slice  nbits=16  boolean_output=off  mode=Upper Bit Location + Width  bit1=0  base1=MSB of Input  bit0=0  base0=LSB of Input  dbl_ovrd=off  block_type=slice
  c_to_ri : casper_library_misc/c_to_ri  n_bits=8  bin_pt=7
      settings: AttributesFormatString=8_7 r/i  SourceProductName=CASPER DSP Blockset
  ri_to_c : casper_library_misc/ri_to_c
      settings: SourceProductName=CASPER DSP Blockset
  Out1 : Outport
  wires:
  c_to_ri/2 -> Slice2/1
  ri_to_c/1 -> Out1/1
  c_to_ri/1 -> Slice1/1
  Slice2/1 -> ri_to_c/2
  In1/1 -> c_to_ri/1
  Slice1/1 -> ri_to_c/1

== system fft_test/slice26 ==
  In1 : Inport
  Slice1 : xbsIndex_r4/Slice  nbits=16  boolean_output=off  mode=Upper Bit Location + Width  bit1=0  base1=MSB of Input  bit0=0  base0=LSB of Input  dbl_ovrd=off  block_type=slice
  Slice2 : xbsIndex_r4/Slice  nbits=16  boolean_output=off  mode=Upper Bit Location + Width  bit1=0  base1=MSB of Input  bit0=0  base0=LSB of Input  dbl_ovrd=off  block_type=slice
  c_to_ri : casper_library_misc/c_to_ri  n_bits=8  bin_pt=7
      settings: AttributesFormatString=8_7 r/i  SourceProductName=CASPER DSP Blockset
  ri_to_c : casper_library_misc/ri_to_c
      settings: SourceProductName=CASPER DSP Blockset
  Out1 : Outport
  wires:
  Slice1/1 -> ri_to_c/1
  In1/1 -> c_to_ri/1
  Slice2/1 -> ri_to_c/2
  c_to_ri/1 -> Slice1/1
  ri_to_c/1 -> Out1/1
  c_to_ri/2 -> Slice2/1

== system fft_test/slice27 ==
  In1 : Inport
  Slice1 : xbsIndex_r4/Slice  nbits=16  boolean_output=off  mode=Upper Bit Location + Width  bit1=0  base1=MSB of Input  bit0=0  base0=LSB of Input  dbl_ovrd=off  block_type=slice
  Slice2 : xbsIndex_r4/Slice  nbits=16  boolean_output=off  mode=Upper Bit Location + Width  bit1=0  base1=MSB of Input  bit0=0  base0=LSB of Input  dbl_ovrd=off  block_type=slice
  c_to_ri : casper_library_misc/c_to_ri  n_bits=8  bin_pt=7
      settings: AttributesFormatString=8_7 r/i  SourceProductName=CASPER DSP Blockset
  ri_to_c : casper_library_misc/ri_to_c
      settings: SourceProductName=CASPER DSP Blockset
  Out1 : Outport
  wires:
  c_to_ri/2 -> Slice2/1
  ri_to_c/1 -> Out1/1
  c_to_ri/1 -> Slice1/1
  Slice2/1 -> ri_to_c/2
  In1/1 -> c_to_ri/1
  Slice1/1 -> ri_to_c/1

== system fft_test/slice28 ==
  In1 : Inport
  Slice1 : xbsIndex_r4/Slice  nbits=16  boolean_output=off  mode=Upper Bit Location + Width  bit1=0  base1=MSB of Input  bit0=0  base0=LSB of Input  dbl_ovrd=off  block_type=slice
  Slice2 : xbsIndex_r4/Slice  nbits=16  boolean_output=off  mode=Upper Bit Location + Width  bit1=0  base1=MSB of Input  bit0=0  base0=LSB of Input  dbl_ovrd=off  block_type=slice
  c_to_ri : casper_library_misc/c_to_ri  n_bits=8  bin_pt=7
      settings: AttributesFormatString=8_7 r/i  SourceProductName=CASPER DSP Blockset
  ri_to_c : casper_library_misc/ri_to_c
      settings: SourceProductName=CASPER DSP Blockset
  Out1 : Outport
  wires:
  c_to_ri/2 -> Slice2/1
  ri_to_c/1 -> Out1/1
  c_to_ri/1 -> Slice1/1
  Slice2/1 -> ri_to_c/2
  In1/1 -> c_to_ri/1
  Slice1/1 -> ri_to_c/1

== system fft_test/slice29 ==
  In1 : Inport
  Slice1 : xbsIndex_r4/Slice  nbits=16  boolean_output=off  mode=Upper Bit Location + Width  bit1=0  base1=MSB of Input  bit0=0  base0=LSB of Input  dbl_ovrd=off  block_type=slice
  Slice2 : xbsIndex_r4/Slice  nbits=16  boolean_output=off  mode=Upper Bit Location + Width  bit1=0  base1=MSB of Input  bit0=0  base0=LSB of Input  dbl_ovrd=off  block_type=slice
  c_to_ri : casper_library_misc/c_to_ri  n_bits=8  bin_pt=7
      settings: AttributesFormatString=8_7 r/i  SourceProductName=CASPER DSP Blockset
  ri_to_c : casper_library_misc/ri_to_c
      settings: SourceProductName=CASPER DSP Blockset
  Out1 : Outport
  wires:
  Slice1/1 -> ri_to_c/1
  In1/1 -> c_to_ri/1
  Slice2/1 -> ri_to_c/2
  c_to_ri/1 -> Slice1/1
  ri_to_c/1 -> Out1/1
  c_to_ri/2 -> Slice2/1

== system fft_test/slice3 ==
  In1 : Inport
  Slice1 : xbsIndex_r4/Slice  nbits=16  boolean_output=off  mode=Upper Bit Location + Width  bit1=0  base1=MSB of Input  bit0=0  base0=LSB of Input  dbl_ovrd=off  block_type=slice
  Slice2 : xbsIndex_r4/Slice  nbits=16  boolean_output=off  mode=Upper Bit Location + Width  bit1=0  base1=MSB of Input  bit0=0  base0=LSB of Input  dbl_ovrd=off  block_type=slice
  c_to_ri : casper_library_misc/c_to_ri  n_bits=8  bin_pt=7
      settings: AttributesFormatString=8_7 r/i  SourceProductName=CASPER DSP Blockset
  ri_to_c : casper_library_misc/ri_to_c
      settings: SourceProductName=CASPER DSP Blockset
  Out1 : Outport
  wires:
  Slice1/1 -> ri_to_c/1
  In1/1 -> c_to_ri/1
  Slice2/1 -> ri_to_c/2
  c_to_ri/1 -> Slice1/1
  ri_to_c/1 -> Out1/1
  c_to_ri/2 -> Slice2/1

== system fft_test/slice30 ==
  In1 : Inport
  Slice1 : xbsIndex_r4/Slice  nbits=16  boolean_output=off  mode=Upper Bit Location + Width  bit1=0  base1=MSB of Input  bit0=0  base0=LSB of Input  dbl_ovrd=off  block_type=slice
  Slice2 : xbsIndex_r4/Slice  nbits=16  boolean_output=off  mode=Upper Bit Location + Width  bit1=0  base1=MSB of Input  bit0=0  base0=LSB of Input  dbl_ovrd=off  block_type=slice
  c_to_ri : casper_library_misc/c_to_ri  n_bits=8  bin_pt=7
      settings: AttributesFormatString=8_7 r/i  SourceProductName=CASPER DSP Blockset
  ri_to_c : casper_library_misc/ri_to_c
      settings: SourceProductName=CASPER DSP Blockset
  Out1 : Outport
  wires:
  Slice1/1 -> ri_to_c/1
  In1/1 -> c_to_ri/1
  Slice2/1 -> ri_to_c/2
  c_to_ri/1 -> Slice1/1
  ri_to_c/1 -> Out1/1
  c_to_ri/2 -> Slice2/1

== system fft_test/slice31 ==
  In1 : Inport
  Slice1 : xbsIndex_r4/Slice  nbits=16  boolean_output=off  mode=Upper Bit Location + Width  bit1=0  base1=MSB of Input  bit0=0  base0=LSB of Input  dbl_ovrd=off  block_type=slice
  Slice2 : xbsIndex_r4/Slice  nbits=16  boolean_output=off  mode=Upper Bit Location + Width  bit1=0  base1=MSB of Input  bit0=0  base0=LSB of Input  dbl_ovrd=off  block_type=slice
  c_to_ri : casper_library_misc/c_to_ri  n_bits=8  bin_pt=7
      settings: AttributesFormatString=8_7 r/i  SourceProductName=CASPER DSP Blockset
  ri_to_c : casper_library_misc/ri_to_c
      settings: SourceProductName=CASPER DSP Blockset
  Out1 : Outport
  wires:
  c_to_ri/2 -> Slice2/1
  ri_to_c/1 -> Out1/1
  c_to_ri/1 -> Slice1/1
  Slice2/1 -> ri_to_c/2
  In1/1 -> c_to_ri/1
  Slice1/1 -> ri_to_c/1

== system fft_test/slice4 ==
  In1 : Inport
  Slice1 : xbsIndex_r4/Slice  nbits=16  boolean_output=off  mode=Upper Bit Location + Width  bit1=0  base1=MSB of Input  bit0=0  base0=LSB of Input  dbl_ovrd=off  block_type=slice
  Slice2 : xbsIndex_r4/Slice  nbits=16  boolean_output=off  mode=Upper Bit Location + Width  bit1=0  base1=MSB of Input  bit0=0  base0=LSB of Input  dbl_ovrd=off  block_type=slice
  c_to_ri : casper_library_misc/c_to_ri  n_bits=8  bin_pt=7
      settings: AttributesFormatString=8_7 r/i  SourceProductName=CASPER DSP Blockset
  ri_to_c : casper_library_misc/ri_to_c
      settings: SourceProductName=CASPER DSP Blockset
  Out1 : Outport
  wires:
  c_to_ri/2 -> Slice2/1
  ri_to_c/1 -> Out1/1
  c_to_ri/1 -> Slice1/1
  Slice2/1 -> ri_to_c/2
  In1/1 -> c_to_ri/1
  Slice1/1 -> ri_to_c/1

== system fft_test/slice5 ==
  In1 : Inport
  Slice1 : xbsIndex_r4/Slice  nbits=16  boolean_output=off  mode=Upper Bit Location + Width  bit1=0  base1=MSB of Input  bit0=0  base0=LSB of Input  dbl_ovrd=off  block_type=slice
  Slice2 : xbsIndex_r4/Slice  nbits=16  boolean_output=off  mode=Upper Bit Location + Width  bit1=0  base1=MSB of Input  bit0=0  base0=LSB of Input  dbl_ovrd=off  block_type=slice
  c_to_ri : casper_library_misc/c_to_ri  n_bits=8  bin_pt=7
      settings: AttributesFormatString=8_7 r/i  SourceProductName=CASPER DSP Blockset
  ri_to_c : casper_library_misc/ri_to_c
      settings: SourceProductName=CASPER DSP Blockset
  Out1 : Outport
  wires:
  Slice1/1 -> ri_to_c/1
  In1/1 -> c_to_ri/1
  Slice2/1 -> ri_to_c/2
  c_to_ri/1 -> Slice1/1
  ri_to_c/1 -> Out1/1
  c_to_ri/2 -> Slice2/1

== system fft_test/slice6 ==
  In1 : Inport
  Slice1 : xbsIndex_r4/Slice  nbits=16  boolean_output=off  mode=Upper Bit Location + Width  bit1=0  base1=MSB of Input  bit0=0  base0=LSB of Input  dbl_ovrd=off  block_type=slice
  Slice2 : xbsIndex_r4/Slice  nbits=16  boolean_output=off  mode=Upper Bit Location + Width  bit1=0  base1=MSB of Input  bit0=0  base0=LSB of Input  dbl_ovrd=off  block_type=slice
  c_to_ri : casper_library_misc/c_to_ri  n_bits=8  bin_pt=7
      settings: AttributesFormatString=8_7 r/i  SourceProductName=CASPER DSP Blockset
  ri_to_c : casper_library_misc/ri_to_c
      settings: SourceProductName=CASPER DSP Blockset
  Out1 : Outport
  wires:
  Slice1/1 -> ri_to_c/1
  In1/1 -> c_to_ri/1
  Slice2/1 -> ri_to_c/2
  c_to_ri/1 -> Slice1/1
  ri_to_c/1 -> Out1/1
  c_to_ri/2 -> Slice2/1

== system fft_test/slice7 ==
  In1 : Inport
  Slice1 : xbsIndex_r4/Slice  nbits=16  boolean_output=off  mode=Upper Bit Location + Width  bit1=0  base1=MSB of Input  bit0=0  base0=LSB of Input  dbl_ovrd=off  block_type=slice
  Slice2 : xbsIndex_r4/Slice  nbits=16  boolean_output=off  mode=Upper Bit Location + Width  bit1=0  base1=MSB of Input  bit0=0  base0=LSB of Input  dbl_ovrd=off  block_type=slice
  c_to_ri : casper_library_misc/c_to_ri  n_bits=8  bin_pt=7
      settings: AttributesFormatString=8_7 r/i  SourceProductName=CASPER DSP Blockset
  ri_to_c : casper_library_misc/ri_to_c
      settings: SourceProductName=CASPER DSP Blockset
  Out1 : Outport
  wires:
  c_to_ri/2 -> Slice2/1
  ri_to_c/1 -> Out1/1
  c_to_ri/1 -> Slice1/1
  Slice2/1 -> ri_to_c/2
  In1/1 -> c_to_ri/1
  Slice1/1 -> ri_to_c/1

== system fft_test/slice8 ==
  In1 : Inport
  Slice1 : xbsIndex_r4/Slice  nbits=16  boolean_output=off  mode=Upper Bit Location + Width  bit1=0  base1=MSB of Input  bit0=0  base0=LSB of Input  dbl_ovrd=off  block_type=slice
  Slice2 : xbsIndex_r4/Slice  nbits=16  boolean_output=off  mode=Upper Bit Location + Width  bit1=0  base1=MSB of Input  bit0=0  base0=LSB of Input  dbl_ovrd=off  block_type=slice
  c_to_ri : casper_library_misc/c_to_ri  n_bits=8  bin_pt=7
      settings: AttributesFormatString=8_7 r/i  SourceProductName=CASPER DSP Blockset
  ri_to_c : casper_library_misc/ri_to_c
      settings: SourceProductName=CASPER DSP Blockset
  Out1 : Outport
  wires:
  c_to_ri/2 -> Slice2/1
  ri_to_c/1 -> Out1/1
  c_to_ri/1 -> Slice1/1
  Slice2/1 -> ri_to_c/2
  In1/1 -> c_to_ri/1
  Slice1/1 -> ri_to_c/1

== system fft_test/slice9 ==
  In1 : Inport
  Slice1 : xbsIndex_r4/Slice  nbits=16  boolean_output=off  mode=Upper Bit Location + Width  bit1=0  base1=MSB of Input  bit0=0  base0=LSB of Input  dbl_ovrd=off  block_type=slice
  Slice2 : xbsIndex_r4/Slice  nbits=16  boolean_output=off  mode=Upper Bit Location + Width  bit1=0  base1=MSB of Input  bit0=0  base0=LSB of Input  dbl_ovrd=off  block_type=slice
  c_to_ri : casper_library_misc/c_to_ri  n_bits=8  bin_pt=7
      settings: AttributesFormatString=8_7 r/i  SourceProductName=CASPER DSP Blockset
  ri_to_c : casper_library_misc/ri_to_c
      settings: SourceProductName=CASPER DSP Blockset
  Out1 : Outport
  wires:
  Slice1/1 -> ri_to_c/1
  In1/1 -> c_to_ri/1
  Slice2/1 -> ri_to_c/2
  c_to_ri/1 -> Slice1/1
  ri_to_c/1 -> Out1/1
  c_to_ri/2 -> Slice2/1
